simulink model "CLIK_PSEUDO_V2"  (R2023a)
settings: Solver=ode1  StartTime=0.0  StopTime=25  FixedStep=Ts  RelTol=1e-3
values from neighbouring files (symbols this model uses):
  Ts = 0.001    [TRAJ.m]
undefined symbols (not defined in the file or in its folder): DiscIntNeverNeededParam
settings Model: Creator=39388  LastModifiedBy=39388

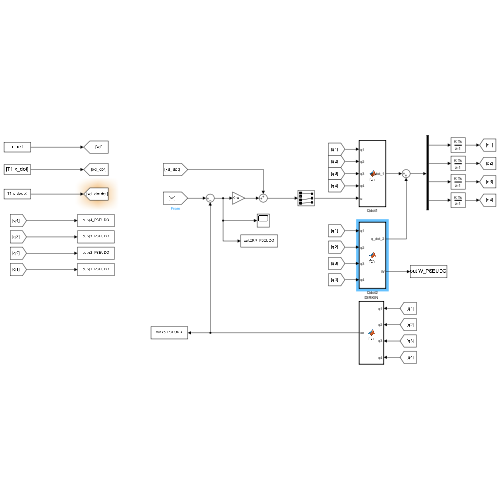
[thumbnail: Simulink's stored preview of the top-level diagram]
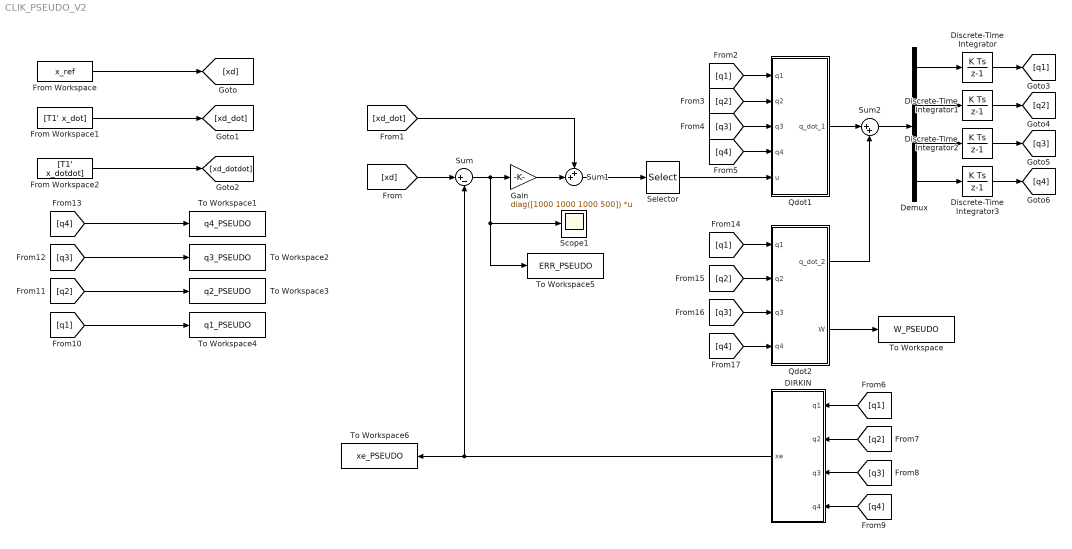
== system CLIK_PSEUDO_V2 ==
  DIRKIN : MATLAB Function  TreatAsAtomicUnit=on
  Demux : Demux
  Discrete-Time Integrator : DiscreteIntegrator  SampleTime=Ts  ICPrevOutput=DiscIntNeverNeededParam  ICPrevScaledInput=DiscIntNeverNeededParam
  Discrete-Time Integrator1 : DiscreteIntegrator  InitialCondition=pi/2  SampleTime=Ts  ICPrevOutput=DiscIntNeverNeededParam  ICPrevScaledInput=DiscIntNeverNeededParam
  Discrete-Time Integrator2 : DiscreteIntegrator  InitialCondition=-0.25  SampleTime=Ts  ICPrevOutput=DiscIntNeverNeededParam  ICPrevScaledInput=DiscIntNeverNeededParam
  Discrete-Time Integrator3 : DiscreteIntegrator  InitialCondition=-pi  SampleTime=Ts  ICPrevOutput=DiscIntNeverNeededParam  ICPrevScaledInput=DiscIntNeverNeededParam
  From Workspace : FromWorkspace  VariableName=x_ref
  From Workspace1 : FromWorkspace  VariableName=[T1' x_dot]
  From Workspace2 : FromWorkspace  VariableName=[T1' x_dotdot]
  Gain : Gain  Gain=diag([1000 1000 1000 500])  Multiplication=Matrix(K*u)
  Qdot1 : MATLAB Function  TreatAsAtomicUnit=on
  Qdot2 : MATLAB Function  TreatAsAtomicUnit=on
  Scope1 : Scope
  Selector : Selector  InputPortWidth=4  IndexOptions=Index vector (dialog)  Indices=[1 3 4]  OutputSizes=1
  Sum : Sum  Inputs=|+-
  Sum1 : Sum  Inputs=++|
  Sum2 : Sum  Inputs=|++
  To Workspace : ToWorkspace  VariableName=W_PSEUDO  SaveFormat=Structure With Time  SampleTime=-1
  To Workspace1 : ToWorkspace  VariableName=q4_PSEUDO  SaveFormat=Structure With Time  SampleTime=-1
  To Workspace2 : ToWorkspace  VariableName=q3_PSEUDO  SaveFormat=Structure With Time  SampleTime=-1
  To Workspace3 : ToWorkspace  VariableName=q2_PSEUDO  SaveFormat=Structure With Time  SampleTime=-1
  To Workspace4 : ToWorkspace  VariableName=q1_PSEUDO  SaveFormat=Structure With Time  SampleTime=-1
  To Workspace5 : ToWorkspace  VariableName=ERR_PSEUDO  SaveFormat=Structure With Time  SampleTime=-1
  To Workspace6 : ToWorkspace  VariableName=xe_PSEUDO  SaveFormat=Structure With Time  SampleTime=-1
  wires:
  From Workspace1/1 -> [xd_dot]
  From Workspace2/1 -> [xd_dotdot]
  [xd] -> Sum/1
  Sum/1 -> To Workspace5/1, Scope1/1, Gain/1
  Gain/1 -> Sum1/2
  [xd_dot] -> Sum1/1
  DIRKIN/1(xe) -> To Workspace6/1, Sum/2
  From Workspace/1 -> [xd]
  Demux/1 -> Discrete-Time Integrator/1
  Demux/2 -> Discrete-Time Integrator1/1
  Demux/3 -> Discrete-Time Integrator2/1
  Demux/4 -> Discrete-Time Integrator3/1
  Discrete-Time Integrator/1 -> [q1]
  Discrete-Time Integrator1/1 -> [q2]
  Discrete-Time Integrator2/1 -> [q3]
  Discrete-Time Integrator3/1 -> [q4]
  [q1] -> Qdot1/1(q1)
  [q2] -> Qdot1/2(q2)
  [q3] -> Qdot1/3(q3)
  [q4] -> Qdot1/4(q4)
  [q1] -> DIRKIN/1(q1)
  [q2] -> DIRKIN/2(q2)
  [q3] -> DIRKIN/3(q3)
  [q4] -> DIRKIN/4(q4)
  [q4] -> To Workspace1/1
  [q3] -> To Workspace2/1
  [q2] -> To Workspace3/1
  [q1] -> To Workspace4/1
  Qdot1/1(q_dot_1) -> Sum2/1
  Sum2/1 -> Demux/1
  [q2] -> Qdot2/2(q2)
  [q1] -> Qdot2/1(q1)
  [q3] -> Qdot2/3(q3)
  [q4] -> Qdot2/4(q4)
  Qdot2/1(q_dot_2) -> Sum2/2
  Qdot2/2(W) -> To Workspace/1
  Selector/1 -> Qdot1/5(u)
  Sum1/1 -> Selector/1

== matlab function CLIK_PSEUDO_V2/DIRKIN ==
  data: q1 input; xe output; q2 input; q3 input; q4 input
function xe = fcn(q1,q2,q3,q4)

xe=[0.5*cos(q1)+0.5*cos(q1+q2);
    0.5*sin(q1)+0.5*sin(q1+q2);
    1+q3;
    q1+q2+q4];

== matlab function CLIK_PSEUDO_V2/Qdot1 ==
  data: q1 input; q2 input; q3 input; q4 input; u input; q_dot_1 output
function  q_dot_1 = fcn(q1,q2,q3,q4,u)

    Jr=[-0.5*sin(q1-0.5*sin(q1+q2)) -0.5*sin(q1+q2) 0 0;
        0                               0                 1 0;
        1                               1                 0 1];

     q_dot_1=Jr'*inv(Jr*Jr')*u;

== matlab function CLIK_PSEUDO_V2/Qdot2 ==
  data: q1 input; q2 input; q3 input; q4 input; q_dot_2 output; W output
function  [q_dot_2,W] = fcn(q1,q2,q3,q4)

    Jr=[-0.5*sin(q1-0.5*sin(q1+q2)) -0.5*sin(q1+q2) 0 0;
        0                               0                 1 0;
        1                               1                 0 1];

    K0=eye(4)*10;

    q_dot_0=K0*[0; 0.25*sin(q2)*cos(q2)/abs(sin(q2)); 0; 0];

    q_dot_2=(eye(4)-Jr'*inv(Jr*Jr')*Jr)*q_dot_0;
    W=0.25*abs(sin(q2));
